simulink model "DAB_OL_loss_cal"  (R2023b)
settings: Solver=VariableStepAuto  StartTime=0.0  StopTime=0.5  RelTol=1e-3
undefined symbols (not defined in the file): Ion, Lithium
libraries: spsMosfetLib x8, spsMeanLib x6, spsVoltageMeasurementLib x6, spsCurrentMeasurementLib x4, spsSeriesRLCBranchLib x4, spsBatteryLib x1, spsDCVoltageSourceLib x1, spsLinearTransformerLib x1, spsRMSLib x1, eeGeneralControl x1, spspowerguiLib x1
settings Model: Creator=Project_Account  LastModifiedBy=saswa
settings ModelReferenceCC: EnableRefExpFcnMdlSchedulingChecks=on

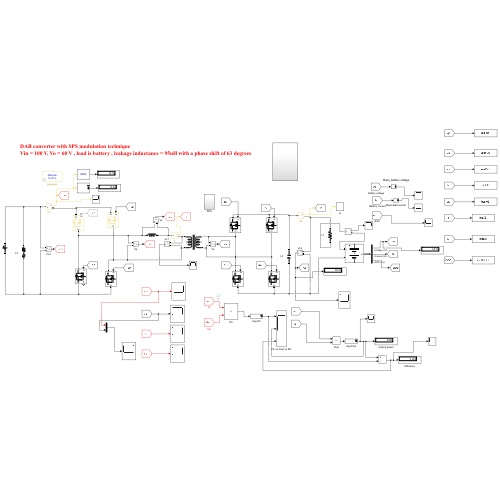
[thumbnail: Simulink's stored preview of the top-level diagram]
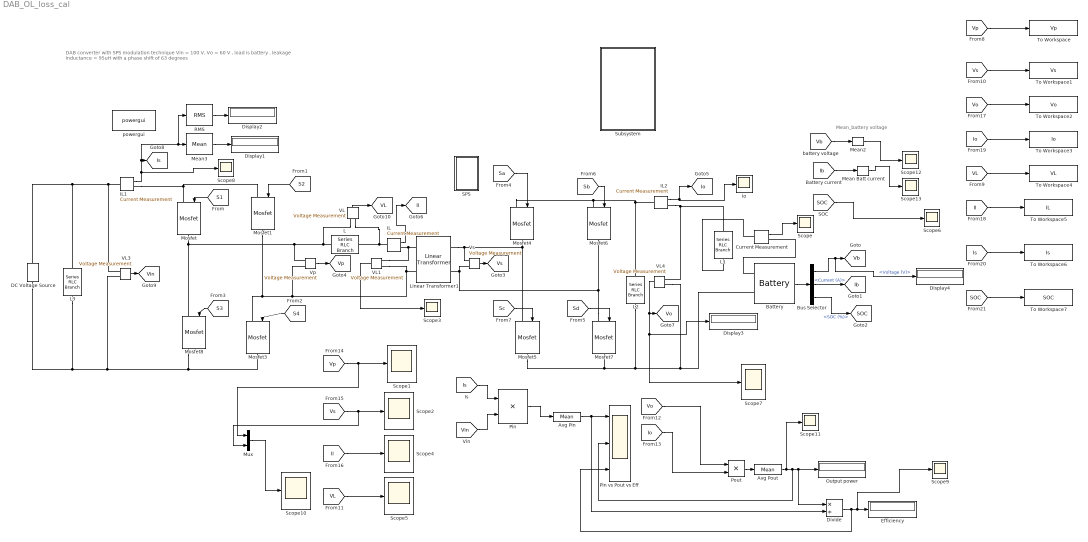
== system DAB_OL_loss_cal ==
  note: Mean_battery voltage
  note: DAB converter with SPS modulation technique
      | Vin = 100 V, Vo = 60 V , load is battery , leakage inductance = 95uH with a phase shift of 63 degrees
  Avg Pin : spsMeanLib/Mean  Freq=50000  Vinit=0  Ts=1e-7
  Avg Pout : spsMeanLib/Mean  Freq=50000  Vinit=0  Ts=1e-7
  Battery : spsBatteryLib/Battery  BatType=Lithium-Ion  ShowTempParam=off  ThermalPreset=no  ShowAgeParam=off  NomV=60  NomQ=120  SOC=60  Batt_Tr=0.1  PresetModel=on  MaxQ=120  MinV=45  FullV=69.8392  Dis_rate=52.1739  R=0.005  Normal_OP=108.5217  expZone="[64.8232      5.89565]"  current=[6.5 13 32.5]  Units=Time  Tci=20  NomT=20  T2=-30  MaxQ2=4.8  FullV2=7.1  Normal_OP2=5.655  expZone2="[6.58           1]"  Rca=0.6  ti=2000  Dp=0  Neq0=0  Tsim=1e6  Ta1=25  Qeol=5.4*0.9  Reol=0.013333*1.2  Char_age=[2.3478, 3]  Dis_age=[2.3478, 10]  N1=1500  N2=10500  N3=1000  N4=1400  Ta2=45  N5=950
  Bus Selector : BusSelector  OutputSignals=Voltage (V),Current (A),SOC (%)
  Current Measurement : spsCurrentMeasurementLib/Current Measurement  PhasorSimulation=off  OutputType=Complex  PSBequivalent=0
  DC Voltage Source : spsDCVoltageSourceLib/DC Voltage Source  Amplitude=400  Measurements=None
  Display{1..4} (4 alike) : Display
  Divide : Product  Inputs=*/
  Efficiency : Display
  IL : spsCurrentMeasurementLib/Current Measurement  PhasorSimulation=off  OutputType=Complex  PSBequivalent=0
  IL1 : spsCurrentMeasurementLib/Current Measurement  PhasorSimulation=off  OutputType=Complex  PSBequivalent=0
  IL2 : spsCurrentMeasurementLib/Current Measurement  PhasorSimulation=off  OutputType=Complex  PSBequivalent=0
  Io : Scope
  L : spsSeriesRLCBranchLib/Series RLC Branch  LConnTagsString=__new0  RConnTagsString=__new0  BranchType=L  Resistance=1  Inductance=95e-6  SetiL0=off  InitialCurrent=0  Capacitance=1e-6  Setx0=off  InitialVoltage=0  Measurements=None
  L1 : spsSeriesRLCBranchLib/Series RLC Branch  LConnTagsString=__new0  RConnTagsString=__new0  BranchType=R  Resistance=0.01  Inductance=19.108e-6*2  SetiL0=off  InitialCurrent=0  Capacitance=1000e-6  Setx0=off  InitialVoltage=0  Measurements=None
  L2 : spsSeriesRLCBranchLib/Series RLC Branch  LConnTagsString=__new0  RConnTagsString=__new0  BranchType=C  Resistance=0.8  Inductance=19.108e-6*2  SetiL0=off  InitialCurrent=0  Capacitance=1200e-6  Setx0=off  InitialVoltage=0  Measurements=None
  L3 : spsSeriesRLCBranchLib/Series RLC Branch  LConnTagsString=__new0  RConnTagsString=__new0  BranchType=RC  Resistance=0.8  Inductance=19.108e-6*2  SetiL0=off  InitialCurrent=0  Capacitance=1200e-6  Setx0=off  InitialVoltage=0  Measurements=None
  Linear Transformer1 : spsLinearTransformerLib/Linear Transformer  UNITS=SI  NominalPower=[1500 50000 ]  winding1=[400 0 0]  winding2=[60 0 0]  ThreeWindings=off  winding3=[3.15e+05 0.7938 0.084225]  RmLm=[5000 5866]  Measurements=None  DataType=on
  Mean Batt current : spsMeanLib/Mean  Freq=20000  Vinit=0  Ts=1e-7
  Mean2 : spsMeanLib/Mean  Freq=20000  Vinit=0  Ts=1e-7
  Mean3 : spsMeanLib/Mean  Freq=15000  Vinit=0  Ts=1e-6
  Mosfet{,1,3..7} (7 alike) : spsMosfetLib/Mosfet  Ron=0.01  Lon=0  Rd=0.01  Vfd=0  IC=0  Rs=1e5  Cs=inf  Measurements=off
  Mosfet8 : spsMosfetLib/Mosfet  Ron=0.01  Lon=0  Rd=0.01  Vfd=0  IC=0  Rs=1e5  Cs=inf  Measurements=on
  Mux : Mux  Inputs=2
  Output power : Display
  Pin : Product
  "Pin vs Pout vs Eff " : Scope  NumInputPorts=3
  Pout : Product
  RMS : spsRMSLib/RMS  TrueRMS=on  Freq=60  RMSInit=120  Ts=0
  SPS : Subsystem
  Scope{,1..13} (14 alike) : Scope
  Subsystem : Subsystem
  To Workspace : ToWorkspace  VariableName=Vp  SaveFormat=Structure With Time  SampleTime=-1
  To Workspace1 : ToWorkspace  VariableName=Vs  SaveFormat=Structure  SampleTime=-1
  To Workspace2 : ToWorkspace  VariableName=Vo  SaveFormat=Structure  SampleTime=-1
  To Workspace3 : ToWorkspace  VariableName=Io  SaveFormat=Structure  SampleTime=-1
  To Workspace4 : ToWorkspace  VariableName=VL  SaveFormat=Structure  SampleTime=-1
  To Workspace5 : ToWorkspace  VariableName=IL  SaveFormat=Structure  SampleTime=-1
  To Workspace6 : ToWorkspace  VariableName=Is  SaveFormat=Structure  SampleTime=-1
  To Workspace7 : ToWorkspace  VariableName=SOC  SaveFormat=Structure  SampleTime=-1
  VL{,1,3..4} (4 alike) : spsVoltageMeasurementLib/Voltage Measurement  PhasorSimulation=off  OutputType=Complex  PSBequivalent=0
  Vp : spsVoltageMeasurementLib/Voltage Measurement  PhasorSimulation=off  OutputType=Complex  PSBequivalent=0
  Vs : spsVoltageMeasurementLib/Voltage Measurement  PhasorSimulation=off  OutputType=Complex  PSBequivalent=0
  powergui : spspowerguiLib/powergui  Priority=1  SimulationMode=Discrete  SampleTime=1e-7  frequency=60  Iterations=50  frequencyindice=0  Pbase=100e6  ErrMax=1e-4  UnitsV=kV  UnitsW=MW  buscounter=0  FunctionMessages=off  echomessages=off  EnableUseOfTLC=off  CurrentSourceSwitches=off  DisableSnubberDevices=off  DisableRonSwitches=off  DisableVfSwitches=off  DisplayEquations=off  AutomaticDiscreteSolvers=off  SolverType=Tustin/Backward Euler (TBE)  Interpol=off  ExternalGateDelay=off  methode=off  Ts=100  x0status=blocks  SPID=on  SwTol=0  HookPort=off  NonlinearTolerance=1e-6  nMaxIteration=1000  ContinueOnMaxIteration=off  RestoreLinks=warning  ResistiveCurrentMeasurement=off  Frange=[0:2:500]  Ylog=off  Xlog=on  ShowGrid=off  save=off  variable=ZData  structure=0  ZoomFFT=off  StartTime=0.0  cycles=1  DisplayStyle=1  fundamental=60  FreqAxis=off  MaxFrequency=1000  frequencyindicesteady=1  RmsSteady=1  display=off
  tag scope: Ib=global, Il=global, Io=global, Is=global, SOC=global, VL=global, Vb=global, Vin=global, Vo=global, Vp=global, Vs=global
  wires:
  VL1/1 -> Scope3/1
  [S3] -> Mosfet8/1
  Mean2/1 -> Scope12/1
  [Sb] -> Mosfet6/1
  [Ib] -> Mean Batt current/1
  [Vb] -> Mean2/1
  [Sc] -> Mosfet5/1
  VL4/1 -> Scope7/1, Display3/1, [Vo]
  [Vin] -> Pin/2
  [Vo] -> Pout/1
  VL/1 -> [VL]
  IL2/1 -> [Io], Io/1
  [S2] -> Mosfet1/1
  VL3/1 -> [Vin]
  [S4] -> Mosfet3/1
  Vp/1 -> [Vp]
  Mean3/1 -> Display1/1
  IL1/1 -> Scope8/1, RMS/1, Mean3/1, [Is]
  Bus Selector/1 -> Display4/1, [Vb]  "<Voltage (V)>"
  [Sd] -> Mosfet7/1
  RMS/1 -> Display2/1
  [Io] -> Pout/2
  Vs/1 -> [Vs]
  Mean Batt current/1 -> Scope13/1
  [SOC] -> Scope6/1
  [S1] -> Mosfet/1
  [Vp] -> Mux/1, Scope1/1
  Bus Selector/2 -> [Ib]  "<Current (A)>"
  IL/1 -> [Il]
  [Sa] -> Mosfet4/1
  Battery/1 -> Bus Selector/1
  Bus Selector/3 -> [SOC]  "<SOC (%)>"
  Avg Pout/1 -> Scope11/1, "Pin vs Pout vs Eff "/2, Divide/1, Output power/1
  Divide/1 -> "Pin vs Pout vs Eff "/3, Scope9/1, Efficiency/1
  Pout/1 -> Avg Pout/1
  Avg Pin/1 -> Divide/2, "Pin vs Pout vs Eff "/1
  Pin/1 -> Avg Pin/1
  [Is] -> Pin/1
  [Vs] -> Mux/2, Scope2/1
  [VL] -> Scope5/1
  [Il] -> Scope4/1
  [Vp] -> To Workspace/1
  [Vs] -> To Workspace1/1
  [Il] -> To Workspace5/1
  [VL] -> To Workspace4/1
  [Io] -> To Workspace3/1
  [Vo] -> To Workspace2/1
  [Is] -> To Workspace6/1
  [SOC] -> To Workspace7/1
  Mux/1 -> Scope10/1
  Current Measurement/1 -> Scope/1
  connections:
  Mosfet7/LConn1 -- Vs/LConn2 -- Linear Transformer1/RConn2 -- Mosfet6/RConn1
  IL/LConn1 -- VL/LConn2 -- L/RConn1
  Linear Transformer1/RConn1 -- Vs/LConn1 -- Mosfet5/LConn1 -- Mosfet4/RConn1
  Vp/LConn2 -- VL1/LConn2 -- Linear Transformer1/LConn2 -- Mosfet3/LConn1 -- Mosfet1/RConn1
  VL1/LConn1 -- Linear Transformer1/LConn1 -- IL/RConn1
  Mosfet3/RConn1 -- Mosfet8/RConn1 -- DC Voltage Source/LConn1 -- L3/RConn1 -- VL3/LConn2
  Mosfet/RConn1 -- Vp/LConn1 -- VL/LConn1 -- L/LConn1 -- Mosfet8/LConn1
  VL3/LConn1 -- IL1/LConn1 -- L3/LConn1 -- DC Voltage Source/RConn1
  Mosfet/LConn1 -- IL1/RConn1 -- Mosfet1/LConn1
  L1/LConn1 -- IL2/RConn1 -- VL4/LConn1
  Mosfet4/LConn1 -- L2/LConn1 -- IL2/LConn1 -- Mosfet6/LConn1
  L2/RConn1 -- Battery/LConn2 -- VL4/LConn2 -- Mosfet7/RConn1 -- Mosfet5/RConn1
  Current Measurement/LConn1 -- L1/RConn1
  Battery/LConn1 -- Current Measurement/RConn1

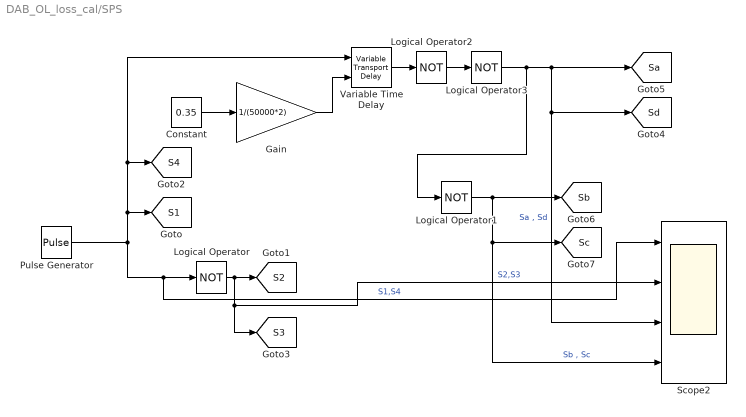
== system DAB_OL_loss_cal/SPS ==
  Constant : Constant  Value=0.35
  Gain : Gain  Gain=1/(50000*2)
  Logical Operator{,1..3} (4 alike) : Logic  Operator=NOT  AllPortsSameDT=off  OutDataTypeStr=boolean
  Pulse Generator : DiscretePulseGenerator  PulseType=Time based  Period=1/50000  PulseWidth=50
  Scope2 : Scope  NumInputPorts=4
  Variable Time Delay : VariableTransportDelay  MaximumDelay=10
  tag scope: S1=global, S2=global, S3=global, S4=global, Sa=global, Sb=global, Sc=global, Sd=global
  wires:
  Variable Time Delay/1 -> Logical Operator2/1
  Logical Operator1/1 -> Scope2/4, [Sc], [Sb]  "Sb , Sc"
  Pulse Generator/1 -> Variable Time Delay/1, [S4], [S1], Scope2/1, Logical Operator/1  "S1,S4"
  Logical Operator/1 -> [S3], Scope2/2, [S2]  "S2,S3"
  Gain/1 -> Variable Time Delay/2
  Constant/1 -> Gain/1
  Logical Operator2/1 -> Logical Operator3/1
  Logical Operator3/1 -> Logical Operator1/1, [Sa], Scope2/3, [Sd]  "Sa , Sd"

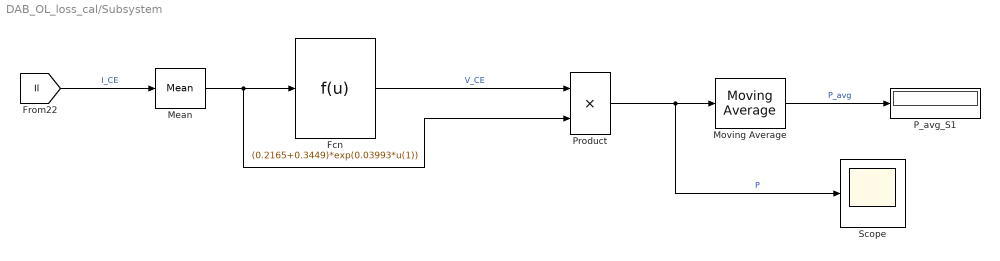
== system DAB_OL_loss_cal/Subsystem ==
  Fcn : Fcn  Expr=(0.2165+0.3449)*exp(0.03993*u(1))
  Mean : spsMeanLib/Mean  Freq=60  Vinit=0  Ts=0
  Moving Average : eeGeneralControl/Moving Average  VariantControl=Variant1  LabelModeActiveChoice=Discrete  f=60  x0=0  BufferSize=8192  Ts=-1
      settings: LibrarySourceBlock=ee_sl_lib/General Control/Moving Average
  P_avg_S1 : Display
  Product : Product
  Scope : Scope
  wires:
  [Il] -> Mean/1  "I_CE"
  Fcn/1 -> Product/1  "V_CE"
  Product/1 -> Scope/1, Moving Average/1  "P"
  Moving Average/1 -> P_avg_S1/1  "P_avg"
  Mean/1 -> Product/2, Fcn/1
